simulink model "Motor_adjust"  (Simulink 7.9)
settings: Solver=ode45  StartTime=0.0  StopTime=0.3  MaxStep=0.0000008  RelTol=1e-8
values from neighbouring files (symbols this model uses):
  J = Jm+J_last/i_getr^2    (= 1.07037741047e-06)    [DC_Motor_RI_Comp.m]
  La = 0*1.792e-3    (= 0)    [DC_Motor_RI_Comp.m]    (also in Sim_Kinematik_Modelle.m = 0.0067; Tol_Kinematik_Modell.m = rnd_vect(n_s,'normal',[La_nom La_tol/3]))
  M_Load = M_last/(i_getr*eta_getr)    (= 0.00103003721425)    [DC_Motor_RI_Comp.m]
  Mo = Io*Psi    (= 0.000558650326277)    [DC_Motor_RI_Comp.m]    (also in Sim_Kinematik_Modelle.m = 0.00152232213911; Tol_Kinematik_Modell.m = Io.*Psi)
  P = 50    [DC_Motor_RI_Comp.m]
  Psi = 1/Ispez    (= 0.0159159637116)    [DC_Motor_RI_Comp.m]    (also in Sim_Kinematik_Modelle.m = 0.0173484004456; Tol_Kinematik_Modell.m = Psi_20*(1+Kemf*(T(T_N)-20)))
  Ra = 6.7    [DC_Motor_RI_Comp.m]    (also in Sim_Kinematik_Modelle.m = 5.1322; Tol_Kinematik_Modell.m = Ra_20*(1+Kr*(T(T_N)-20)))
  Rc = 0.0*Ra    (= 0)    [DC_Motor_RI_Comp.m]    (also in Sim_Kinematik_Modelle.m)
  T_PWM = 1/f_PWM    (= 1.6e-05)    [DC_Motor_RI_Comp.m]    (also in Sim_Kinematik_Modelle.m = 0.005)
  Tc = 0.8*Tm    (= 0.0226483122607)    [DC_Motor_RI_Comp.m]    (also in Sim_Kinematik_Modelle.m = 0.00182524694804)
  Umax = 8*0.8    (= 6.4)    [DC_Motor_RI_Comp.m]
settings Model: Creator=dep02378  LastModifiedBy=dep02378
settings OptimizationCC: InitFltsAndDblsToZero=on
settings DebuggingCC: FcnCallInpInsideContextMsg=Use local settings  StrictBusMsg=Warning
settings GRTTargetCC: CombineOutputUpdateFcns=off  GRTInterface=on

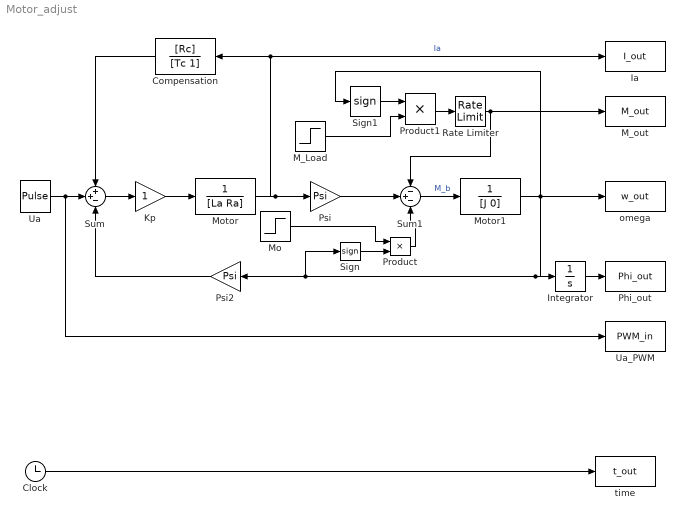
== system Motor_adjust ==
  Clock : Clock
  Compensation : TransferFcn  Numerator=[Rc]  Denominator=[Tc 1]
  Ia : ToWorkspace  VariableName=I_out  SampleTime=-1
  Integrator : Integrator
  Kp : Gain
  M_Load : Step  Time=0.0  After=M_Load  SampleTime=0
  M_out : ToWorkspace  VariableName=M_out  SampleTime=-1
  Mo : Step  Time=0.0  After=Mo  SampleTime=0
  Motor : TransferFcn  Denominator=[La Ra]
  Motor1 : TransferFcn  Denominator=[J 0]
  Phi_out : ToWorkspace  VariableName=Phi_out  SampleTime=-1
  Product : Product  RndMeth=Zero
  Product1 : Product  RndMeth=Zero
  Psi : Gain  Gain=Psi
  Psi2 : Gain  Gain=Psi
  Rate Limiter : RateLimiter  RisingSlewLimit=100  FallingSlewLimit=-100  SampleTimeMode=inherited
  Sign : Signum  ZeroCross=off
  Sign1 : Signum  ZeroCross=off
  Sum : Sum  Inputs=++-
  Sum1 : Sum  Inputs=-+-
  Ua : DiscretePulseGenerator  PulseType=Time based  Amplitude=Umax  Period=T_PWM  PulseWidth=P
  Ua_PWM : ToWorkspace  VariableName=PWM_in  SampleTime=-1
  omega : ToWorkspace  VariableName=w_out  SampleTime=-1
  time : ToWorkspace  VariableName=t_out  SampleTime=-1
  wires:
  Sum/1 -> Kp/1
  Kp/1 -> Motor/1
  Motor/1 -> Psi/1, Compensation/1, Ia/1  "Ia"
  Clock/1 -> time/1
  Sum1/1 -> Motor1/1  "M_b"
  Psi/1 -> Sum1/2
  Psi2/1 -> Sum/3
  Compensation/1 -> Sum/1
  Ua/1 -> Sum/2, Ua_PWM/1
  Integrator/1 -> Phi_out/1
  Sign/1 -> Product/2
  Mo/1 -> Product/1
  Product1/1 -> Rate Limiter/1
  Motor1/1 -> omega/1, Integrator/1, Psi2/1, Sign/1, Sign1/1
  Sign1/1 -> Product1/1
  M_Load/1 -> Product1/2
  Product/1 -> Sum1/3
  Rate Limiter/1 -> M_out/1, Sum1/1
